simulink model "SurroundVehicleSensorFusion"  (R2024b)
settings: Solver=FixedStepAuto  StartTime=0.0  StopTime=10.0  RelTol=1e-3  EnableMultiTasking=on
libraries: trackingutilitieslib x2
settings Model: Creator=The MathWorks, Inc.  LastModifiedBy=The MathWorks, Inc.
settings SolverCC: AlgebraicLoopSolver=TrustRegion  MaxZcPerStep=1
settings DataIOCC: SaveOutput=off
settings OptimizationCC: DefaultParameterBehavior=Inlined  InlineInvariantSignals=on  EnhancedBackFolding=on  PassReuseOutputArgsAs=Individual arguments  ZeroExternalMemoryAtStartup=off  ZeroInternalMemoryAtStartup=off  EfficientFloat2IntCast=on  OptimizeBlockOrder=speed  DifferentSizesBufferReuse=on  OptimizationCustomize=off  EfficientTunableParamExpr=on
settings DebuggingCC: ParameterTunabilityLossMsg=error  UnconnectedInputMsg=warning  UnconnectedOutputMsg=warning  UnconnectedLineMsg=warning  ModelReferenceSymbolNameMessage=none  SubsystemReferenceDiagnosticForUnitTest=warning  IntegerSaturationMsg=none
settings HardwareCC: ProdLongLongMode=on
settings ModelReferenceCC: EnableRefExpFcnMdlSchedulingChecks=on  ModelReferenceNumInstancesAllowed=Single  PropagateVarSize=During execution
settings RTWCC: Description=Embedded Coder  SystemTargetFile=ert.tlc  TemplateMakefile=ert_default_tmf  RTWVerbose=off  BuildConfiguration=Faster Runs  PortableWordSizes=on  CodeExecutionProfiling=on  CodeProfilingSaveOptions=AllData  TargetLang=C++  GPUComputeCapability=3.5  DLArmComputeVersion=19.05
settings CodeAppCC: ForceParamTrailComments=on  IgnoreCustomStorageClasses=off  OperatorAnnotations=on  SimulinkDataObjDesc=on  SFDataObjDesc=on  CustomSymbolStrGlobalVar=$N$M  CustomSymbolStrType=$N$M_T  CustomSymbolStrFcn=APV_$N$M$F  CustomSymbolStrMacro=$N$M  InsertBlockDesc=on
settings ERTTargetCC: TargetLangStandard=C++03 (ISO)  GenerateSampleERTMain=on  CombineSignalStateStructs=on  CodeInterfacePackaging=C++ class  SupportVariableSizeSignals=on  RootIOFormat=Structure reference  ERTCustomFileTemplate=example_file_process.tlc  DynamicArrayContainerType=coder::array

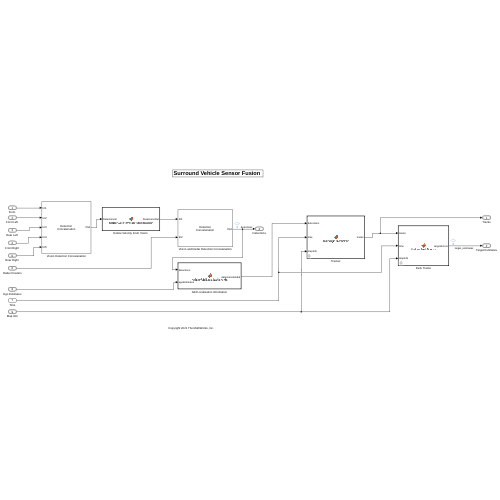
[thumbnail: Simulink's stored preview of the top-level diagram]
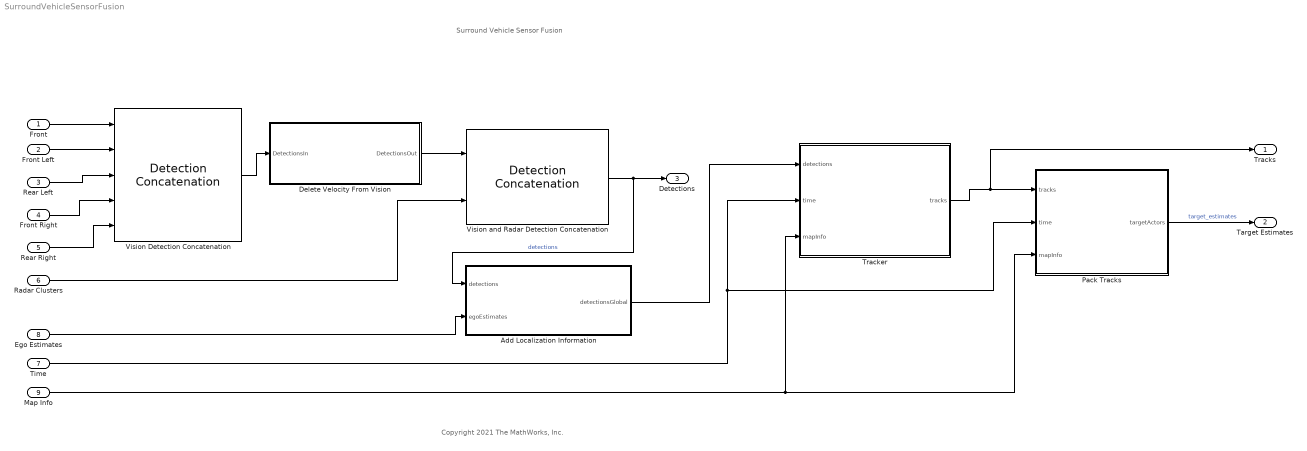
== system SurroundVehicleSensorFusion ==
  note: Copyright 2021 The MathWorks, Inc.
  note: Surround Vehicle Sensor Fusion
  "Front " : Inport  OutDataTypeStr=Bus: BusObjectDetections1  PortDimensions=[1 1]  SampleTime=[0.10000000000000001,0]  BusOutputAsStruct=on
  "Front Left " : Inport  Port=2  OutDataTypeStr=Bus: BusObjectDetections1  PortDimensions=[1 1]  SampleTime=[0.10000000000000001,0]  BusOutputAsStruct=on
  "Rear Left " : Inport  Port=3  OutDataTypeStr=Bus: BusObjectDetections1  PortDimensions=[1 1]  SampleTime=[0.10000000000000001,0]  BusOutputAsStruct=on
  "Front Right " : Inport  Port=4  OutDataTypeStr=Bus: BusObjectDetections1  PortDimensions=[1 1]  SampleTime=[0.10000000000000001,0]  BusOutputAsStruct=on
  "Rear Right " : Inport  Port=5  OutDataTypeStr=Bus: BusObjectDetections1  PortDimensions=[1 1]  SampleTime=[0.10000000000000001,0]  BusOutputAsStruct=on
  Radar Clusters : Inport  Port=6  OutDataTypeStr=Bus: BusDrivingRadarDataGenerator  PortDimensions=[1 1]  SampleTime=[0.10000000000000001,0]  BusOutputAsStruct=on
  Time : Inport  Port=7  OutDataTypeStr=double  PortDimensions=[1 1]  SampleTime=[0.10000000000000001,0]
  Ego Estimates : Inport  Port=8  OutDataTypeStr=Bus: BusEgoPose  PortDimensions=[1 1]  SampleTime=[0.10000000000000001,0]  BusOutputAsStruct=on
  Map Info : Inport  Port=9  OutDataTypeStr=Bus: BusMapInfo  PortDimensions=[1 1]  SampleTime=[0.10000000000000001,0]  BusOutputAsStruct=on
  Add Localization Information : MATLAB Function  Priority=0  TreatAsAtomicUnit=on
  "Delete Velocity From Vision " : MATLAB Function  Priority=0  TreatAsAtomicUnit=on
  Pack Tracks : MATLAB Function  TreatAsAtomicUnit=on  mask{initStruct=Simulink.Bus.createMATLABStruct('BusActorsEgo')}
      mask prompts: initStruct "Output Structure"
  Tracker : MATLAB Function  TreatAsAtomicUnit=on  mask{initStruct=Simulink.Bus.createMATLABStruct('BusTrackerJPDA')}
      mask prompts: initStruct "Output Structure"
  Vision Detection Concatenation : trackingutilitieslib/Detection Concatenation  Priority=0  NumInputs=5  BusNameSource=Auto  BusName=BusConcatenation  SimulateUsing=Interpreted execution
  Vision and Radar Detection Concatenation : trackingutilitieslib/Detection Concatenation  Priority=0  NumInputs=2  BusNameSource=Auto  BusName=BusConcatenation  SimulateUsing=Interpreted execution
  Tracks : Outport  OutDataTypeStr=Bus: BusTrackerJPDA  PortDimensions=[1 1]  SampleTime=[0.10000000000000001,0]  BusOutputAsStruct=on
  Target Estimates : Outport  Port=2  OutDataTypeStr=Bus: BusActorsEgo  PortDimensions=[1 1]  SampleTime=[0.10000000000000001,0]  BusOutputAsStruct=on
  Detections : Outport  Port=3  OutDataTypeStr=Bus: BusDetectionConcatenation2  PortDimensions=[1 1]  SampleTime=[0.10000000000000001,0]  BusOutputAsStruct=on
  wires:
  "Front Left "/1 -> Vision Detection Concatenation/2
  Tracker/1(tracks) -> Tracks/1, Pack Tracks/1(tracks)
  "Delete Velocity From Vision "/1(DetectionsOut) -> Vision and Radar Detection Concatenation/1
  Time/1 -> Pack Tracks/2(time), Tracker/2(time)
  "Front Right "/1 -> Vision Detection Concatenation/4
  Add Localization Information/1(detectionsGlobal) -> Tracker/1(detections)
  Map Info/1 -> Pack Tracks/3(mapInfo), Tracker/3(mapInfo)
  "Rear Right "/1 -> Vision Detection Concatenation/5
  Ego Estimates/1 -> Add Localization Information/2(egoEstimates)
  Vision and Radar Detection Concatenation/1 -> Detections/1, Add Localization Information/1(detections)  "detections"
  "Rear Left "/1 -> Vision Detection Concatenation/3
  Vision Detection Concatenation/1 -> "Delete Velocity From Vision "/1(DetectionsIn)
  "Front "/1 -> Vision Detection Concatenation/1
  Radar Clusters/1 -> Vision and Radar Detection Concatenation/2
  Pack Tracks/1(targetActors) -> Target Estimates/1  "target_estimates"

== matlab function SurroundVehicleSensorFusion/Pack Tracks ==
  data: targetActors output Bus: BusActorsEgo; tracks input; time input; mapInfo input; initStruct parameter
function targetActors = helperPackTracks(tracks,time,mapInfo,initStruct)
targetActors = initStruct; 
numTracks = tracks.NumTracks;
targetActors = initStruct;
targetActors.Time = time;
targetActors.NumActors = numTracks;
targetFrenetStates = zeros(targetActors.NumActors,6);

for i=1:targetActors.NumActors
    s = tracks.Tracks(i,1).State(1);
    ds = tracks.Tracks(i,1).State(2);
    dds = 0;
    d = tracks.Tracks(i,1).State(3);
    dd = tracks.Tracks(i,1).State(4);
    if abs(ds) > 0.5 && abs(dd) > 0.5
        ddbyds = dd./ds;
    else
        ddbyds =0;
    end
    dd2ds2 = 0;
    targetFrenetStates(i,:) = [s;ds;dds;d;ddbyds;dd2ds2];
end

if(targetActors.NumActors)
    globalPlanPoints = mapInfo.GlobalPlanPoints(1:mapInfo.NumGlobalPlanPoints,:); 
    refPathFrenet = referencePathFrenet(globalPlanPoints);  
    targetStates = frenet2global(refPathFrenet, targetFrenetStates);
    for i = 1:targetActors.NumActors      
        targetActors.Actors(i).ActorID = tracks.Tracks(i,1).ObjectAttributes(1,1).TargetIndex;
        tempTargetStates = targetStates(i,:);
        targetActors.Actors(i).Position(1:2) =  tempTargetStates([1 2]);
        speed = tempTargetStates(5);
        theta = tempTargetStates(3);
        targetActors.Actors(i).Velocity(1) =  speed.*cos(theta);
        targetActors.Actors(i).Velocity(2) =  speed.*sin(theta);
        targetActors.Actors(i).Yaw = rad2deg(tempTargetStates(3));
    end
end
end

== matlab function SurroundVehicleSensorFusion/Add Localization Information ==
  data: detections input; detectionsGlobal output Bus: BusConcatenationGlobal; egoEstimates input
function detectionsGlobal = helperAddLocalizationInfo(detections,egoEstimates)
% detections - detections in ego cordinates
% detectionsGlobal - detections in global coordinates

egoPos = egoEstimates.Position(:);
egoVel = egoEstimates.Velocity(:);
egoOrient = egoEstimates.Orientation';
detectionsGlobal.NumDetections = detections.NumDetections;
detectionsGlobal.IsValidTime = detections.IsValidTime;

defaultDetections.Time = detections.Detections(1).Time;
defaultDetections.Measurement = zeros(3,1);
defaultDetections.MeasurementNoise = zeros(3,3);
defaultDetections.SensorIndex      = detections.Detections(1).SensorIndex;
defaultDetections.ObjectClassID      = detections.Detections(1).ObjectClassID;

defaultMeasurementParameters.Frame = detections.Detections(1).MeasurementParameters.Frame;
defaultMeasurementParameters.OriginPosition = detections.Detections(1).MeasurementParameters.OriginPosition;
defaultMeasurementParameters.OriginVelocity = zeros(3,1);
defaultMeasurementParameters.Orientation = detections.Detections(1).MeasurementParameters.Orientation;
defaultMeasurementParameters.HasVelocity = false;
defaultMeasurementParameters.HasElevation = detections.Detections(1).MeasurementParameters.HasElevation;

defaultDetections.MeasurementParameters      = repmat(defaultMeasurementParameters,2,1);
defaultDetections.ObjectAttributes      = detections.Detections(1).ObjectAttributes;
detectionsGlobal.Detections = repmat(defaultDetections,150,1);

sensorToEgo = detectionsGlobal.Detections(1).MeasurementParameters(1,1);
egoParams = detectionsGlobal.Detections(1).MeasurementParameters(1,1);

if detections.NumDetections > 0
    % Add information about egoVehicle to detections to get detectionsGlobal
    for i = 1:detections.NumDetections
        
        % The sensors do not move with respect to ego vehicle
        sensorToEgo.Frame = detections.Detections(i).MeasurementParameters.Frame;
        sensorToEgo.OriginPosition = detections.Detections(i).MeasurementParameters.OriginPosition;
        sensorToEgo.OriginVelocity = zeros(3,1);
        sensorToEgo.Orientation = detections.Detections(i).MeasurementParameters.Orientation;
        sensorToEgo.HasVelocity = detections.Detections(i).MeasurementParameters.HasVelocity;
        sensorToEgo.HasElevation = detections.Detections(i).MeasurementParameters.HasElevation;
        
        % Parameters for scenario to ego transformation
        egoParams.Frame = drivingCoordinateFrameType.Rectangular;
        egoParams.OriginPosition = egoPos;
        egoParams.OriginVelocity = egoVel;
        egoParams.Orientation = egoOrient';
        egoParams.HasVelocity = detections.Detections(i).MeasurementParameters.HasVelocity;
        egoParams.HasElevation = detections.Detections(i).MeasurementParameters.HasElevation;
        
        % Update detectionsGlobal fields using detections
        detectionsGlobal.Detections(i).Time = detections.Detections(i).Time;
        detectionsGlobal.Detections(i).Measurement = detections.Detections(i).Measurement;
        detectionsGlobal.Detections(i).MeasurementNoise = detections.Detections(i).MeasurementNoise;
        detectionsGlobal.Detections(i).SensorIndex = detections.Detections(i).SensorIndex;
        detectionsGlobal.Detections(i).ObjectClassID = 0;
        detectionsGlobal.Detections(i).ObjectAttributes = detections.Detections(i).ObjectAttributes;
        % Update MeasurementParameters of detectionsGlobal
        % using detections in ego coordinates and ego
        % parameters
        detectionsGlobal.Detections(i).MeasurementParameters = [sensorToEgo;egoParams];
        
    end
end
end

== matlab function SurroundVehicleSensorFusion/Delete Velocity From Vision  ==
  data: DetectionsIn input; DetectionsOut output Bus: BusVision
function DetectionsOut = helperDeleteVelocityFromVision(DetectionsIn)
% Construct DetectionsOut and copy values from DetectionsIn
maxReportedDetections = 20;
minMeasurementNoise = 0.0025;
DetectionsOut.NumDetections = DetectionsIn.NumDetections;
DetectionsOut.IsValidTime = DetectionsIn.IsValidTime;
Detections.Time = DetectionsIn.Detections(1).Time;
Detections.Measurement = zeros(3,1);
Detections.MeasurementNoise = zeros(3,3);
Detections.SensorIndex      = DetectionsIn.Detections(1).SensorIndex;
Detections.ObjectClassID      = DetectionsIn.Detections(1).ObjectClassID;
Detections.ObjectAttributes      = DetectionsIn.Detections(1).ObjectAttributes;
Detections.MeasurementParameters      = DetectionsIn.Detections(1).MeasurementParameters;
Detections.MeasurementParameters.HasVelocity      = false; % default should not include velocity
DetectionsOut.Detections = repmat(Detections,maxReportedDetections,1);

if DetectionsOut.NumDetections>0
    for i = 1:DetectionsOut.NumDetections
        DetectionsOut.Detections(i).Measurement = DetectionsIn.Detections(i).Measurement(1:3);
        DetectionsOut.Detections(i).MeasurementNoise = blkdiag(DetectionsIn.Detections(i).MeasurementNoise(1:2,1:2),1/(2*pi));
        DetectionsOut.Detections(i).ObjectClassID      = DetectionsIn.Detections(i).ObjectClassID;
        DetectionsOut.Detections(i).ObjectAttributes.TargetIndex = DetectionsIn.Detections(i).ObjectAttributes.TargetIndex;
        % Add minimum noise to detections for better
        % perfromance of tracker
        if DetectionsOut.Detections(i).MeasurementNoise(1,1) < minMeasurementNoise
            DetectionsOut.Detections(i).MeasurementNoise(1,1)= minMeasurementNoise;
        end
        if DetectionsOut.Detections(i).MeasurementNoise(2,2) < minMeasurementNoise
            DetectionsOut.Detections(i).MeasurementNoise(2,2) = minMeasurementNoise;
        end

        pos = DetectionsOut.Detections(i).Measurement(1:2);
        if abs(pos(1)) < 10  && abs(pos(2)) < 10
            [az, ~, r] = cart2sph(pos(1),pos(2),0);
            [pos(1),pos(2)] = sph2cart(az, 0, r + 1.4); % Increase range
            DetectionsOut.Detections(i).Measurement(1:2) = pos;
            DetectionsOut.Detections(i).MeasurementNoise(1,1) = 2.5;
            DetectionsOut.Detections(i).MeasurementNoise(2,2) = 0.01;
        end

    end
end
end

== matlab function SurroundVehicleSensorFusion/Tracker ==
  data: tracks output Bus: BusTrackerJPDA; detections input; time input; mapInfo input; initStruct parameter
function tracks = helperJPDATracker(detections,time,mapInfo,initStruct)
tracks = initStruct; 
updateReferencePath(mapInfo);

persistent tracker;
persistent firstInstance; 

% Initialize tracker
if (isempty(tracker))
    tracker = trackerJPDA('FilterInitializationFcn',@helperInitRefPathFilter,...
                'AssignmentThreshold',[200 inf],...
                'ConfirmationThreshold',[8 10],...
                'DeletionThreshold',[5 5]);
end

if(isempty(firstInstance))
    firstInstance = true;
end

if(firstInstance)
    if(detections.NumDetections)
         
        numRadarDetections = 0;
        numVisionDetections = 0;
        radarDetections = detections.Detections;
        visionDetections =  detections.Detections;
        for i =1:detections.NumDetections
            if(detections.Detections(i).SensorIndex == 1)
                numRadarDetections = numRadarDetections+1;
                radarDetections(numRadarDetections) = detections.Detections(i);
            else
                numVisionDetections = numVisionDetections+1;
                visionDetections(numVisionDetections) = detections.Detections(i);
            end
        end
        if numRadarDetections
            tracksOut = tracker(radarDetections(1:numRadarDetections), time);
        else
            tracksOut = tracker(visionDetections(1:numVisionDetections), time);
        end
        firstInstance = false;
        tracks = packTracks(tracksOut,initStruct);
    end
else
    for i = 1:detections.NumDetections
        % Add minimum MeasurementNoise for range rate for better
        % perfromance of the tracker
        if(detections.Detections(i).SensorIndex == 1)
            if(detections.Detections(i).MeasurementNoise(3,3) < 2)
                detections.Detections(i).MeasurementNoise(3,3) = 2 ;
            end
            if abs(abs(detections.Detections(i).Measurement(1)) - 24) < 4
                detections.Detections(i).MeasurementNoise(1,1) = max(25, detections.Detections(i).MeasurementNoise(1,1));
            end
        end
    end
    % Invoke tracker 
    tracksOut = tracker(detections.Detections(1:detections.NumDetections), time);
    tracks = packTracks(tracksOut,initStruct);
end
end
function tracks = packTracks(tracksOut,initStruct)
% Pack tracks into a predefined bus with fixed size
tracks = initStruct;
tracks.NumTracks = size(tracksOut,1);
for i=1:tracks.NumTracks
    tracks.Tracks(i).TrackID = tracksOut(i,1).TrackID;
    tracks.Tracks(i).BranchID = tracksOut(i,1).BranchID;
    tracks.Tracks(i).SourceIndex = tracksOut(i,1).SourceIndex;
    tracks.Tracks(i).UpdateTime = tracksOut(i,1).UpdateTime;
    tracks.Tracks(i).Age = tracksOut(i,1).Age;
    tracks.Tracks(i).State = tracksOut(i,1).State;
    tracks.Tracks(i).StateCovariance = tracksOut(i,1).StateCovariance;
    tracks.Tracks(i).ObjectClassID = tracksOut(i,1).ObjectClassID;
    tracks.Tracks(i).TrackLogic = trackLogicType.History;
    tracks.Tracks(i).TrackLogicState = tracksOut(i,1).TrackLogicState;
    tracks.Tracks(i).IsConfirmed = tracksOut(i,1).IsConfirmed;
    tracks.Tracks(i).IsCoasted = tracksOut(i,1).IsCoasted;
    tracks.Tracks(i).IsSelfReported = tracksOut(i,1).IsSelfReported;
    for j=1:size(tracksOut(i,1).ObjectAttributes,2)
        tracks.Tracks(i).ObjectAttributes(j,1) = tracksOut(i,1).ObjectAttributes(1,j);
    end
end
end
function refpath = updateReferencePath(mapInformation)
persistent refpath1;
if(isempty(refpath1))
    if(nargin > 0)
        wp = mapInformation.GlobalPlanPoints(1:mapInformation.NumGlobalPlanPoints,:);
    else
        wp = [0 0;0 1];
    end

    refpath1 = referencePathFrenet(wp);
end
refpath = refpath1;
end
 
function filter = helperInitRefPathFilter(detection)
% This is a helper function used in the object tracking and planning
% example using Frenet coordinates. It may be removed or modified in the
% next release.

% The function defines a constant longitudinal speed and decaying lateral
% speed motion for objects.

% Use initcvekf to convert from measurement space to Cartesian coordinate
% space.
filterCart = initcvekf(detection);

% Convert the state to Frenet coordinates
state = cartToFilterState(filterCart.State);

% Define state covariance
stateCov = blkdiag(5,100,4,5);

% Define filter
filter = trackingEKF(@stateTransFcn,@measurementFcn,state,...
    'StateTransitionJacobianFcn',@stateTransJacobianFcn,...
    'StateCovariance',stateCov,...
    'MeasurementNoise',detection.MeasurementNoise,...
    'HasAdditiveProcessNoise',false,...
    'ProcessNoise',blkdiag(10,1));
end

function state = stateTransFcn(state, wt, dT)
if isscalar(wt)
    w = repmat(wt,[4 size(state,2)]);
else
    w = wt;
end
tau = 3;
state(1,:) = state(1,:) + state(2,:)*dT + w(1,:)*dT^2/2;
state(2,:) = state(2,:) + w(1,:)*dT;
state(3,:) = state(3,:) + state(4,:)*tau*(1 - exp(-dT/tau)) + w(2,:)*dT^2/2;
state(4,:) = state(4,:)*exp(-dT/tau) + w(2,:)*dT;
end

function [dfdx, dfdw] = stateTransJacobianFcn(~, ~, dT)
tau = 3;
dfdx = [1 dT 0 0;0 1 0 0;0 0 1 tau*(1 - exp(-dT/tau));0 0 0 exp(-dT/tau)];
dfdw = [dT^2/2 0;dT 0;0 dT^2/2;0 dT];
end

function z = measurementFcn(x, varargin)
cartState = filterToCartState(x);
z = cvmeas(cartState,varargin{:});
end

function filterState = cartToFilterState(cartState)

% Assemble as global state to use global2frenet
numStates = size(cartState,2);
x = cartState(1,:);
y = cartState(3,:);
theta = atan2(cartState(4,:),cartState(2,:));
speed = sqrt(cartState(4,:).^2 + cartState(2,:).^2);
theta(speed <= 2) = 0;
kappa = zeros(1,numStates);
accel = zeros(1,numStates);
globalState = [x;y;theta;kappa;speed;accel];

% Convert to Frenet state
refPath = updateReferencePath();
refPoint = closestPoint(refPath,[x y]);
deltaTheta = abs(angdiff(refPoint(3),globalState(3)));
if deltaTheta  < pi/2
    frenetState = global2frenet(refPath,globalState')';
else
    globalState(3) = globalState(3) + pi;
    frenetState = global2frenet(refPath,globalState')';
end

% Convert to filter state
s = frenetState(1,:);
ds = frenetState(2,:);
d = frenetState(4,:);
dd = frenetState(5,:).*ds;
filterState = [s;ds;d;dd];
end

function cartState = filterToCartState(filterState)
% Assemble as Frenet state to use frenet2global
numStates = size(filterState,2);
s = filterState(1,:);
ds = filterState(2,:);
dds = zeros(1,numStates);
d = filterState(3,:);
dd = filterState(4,:);
ddbyds = zeros(1,numStates);
ddbyds(abs(ds) > 0.5) = dd(abs(ds) > 0.5)./ds(abs(ds) > 0.5);
dd2ds2 = zeros(1,numStates);
frenetState = [s;ds;dds;d;ddbyds;dd2ds2];

% Convert to global state
refPath = updateReferencePath();
globalState = frenet2global(refPath,frenetState')';

% Convert to cartesian state
x = globalState(1,:);
y = globalState(2,:);
speed = globalState(5,:);
theta = globalState(3,:);
vx = speed.*cos(theta);
vy = speed.*sin(theta);
cartState = [x;vx;y;vy];

end
